simulink model "METI_Thermal_ver01_Jmaab_2018b_Intg"  (R2018b)
settings: Solver=ode8  StartTime=0  StopTime=end_time  FixedStep=sampling_time  RelTol=1e-3
PreLoadFcn:
  | %init_setting;
values from neighbouring files (symbols this model uses):
  degC2K = 273.15    [METI_TRAMI_Thermal_ver01_Jmaab_PreLoad.m]    (also in init_setting_METI.m)
  K2degC = -273.15    [METI_TRAMI_Thermal_ver01_Jmaab_PreLoad.m]    (also in init_setting_METI.m)
  sampling_time = 0.0025    [METI_TRAMI_Thermal_ver01_Jmaab_PreLoad.m]
undefined symbols (not defined in the file or in its folder): ACC_D_Gain, ACC_I_Gain, ACC_P_Gain, ALT_CNT_ALT_OFF_RPM_HYS_rpm, ALT_CNT_ALT_ON_RPM_HYS_rpm, ALT_CNT_Alter_V_BASE_V, ALT_CNT_Alter_V_Kaisei_V, ALT_CNT_flag_disable_kaisei, ALT_CNT_V_Battely_Kudo_V, ALT_PNT_ALT_GDCurrent_A, ALT_PNT_ALT_GDVolt_V, ALT_PNT_Alter_limit_Current_V_table, ALT_PNT_Alter_limit_Current_V_table_x_rpm, ALT_PNT_Alter_trq_Nm_map, ALT_PNT_Alter_trq_Nm_map_x_rpm, ALT_PNT_Alter_trq_Nm_map_y_Current_A, ALT_PNT_Alter_trq_Nm_map_z_Volt_tgt_V, ALT_PNT_eta_pulley_alt, ALT_PNT_Gain_Alt_v_del, ALT_PNT_ratio_pulley_alt, ALT_PNT_Tau_Alternator_V_tgt_s, ALT_PNT_trq_alter_output_LL_Nm, BK_PNT_Pow_UL, BK_PNT_Tau_brake, Brk_LL, Brk_PGain, Brk_UL, BT_PNT_Lo_Capa_lo_batt_F, BT_PNT_Lo_ocv_SOC_lo_batt_OCV_V_table, BT_PNT_Lo_ocv_SOC_lo_batt_OCV_V_table_x_SOC, BT_PNT_Lo_R_lo_batt_ohm, BT_PNT_Lo_SOC_MAX_lo_batt, BT_PNT_Lo_SOC_MIN_lo_batt, BT_PNT_Lo_SOC_START_lo_batt, BT_PNT_Lo_V_start_ocv, DF_PNT_DF_gear, DF_PNT_DFBlock2DFAir_Heat_Resi_KpW, DF_PNT_DFBlock_Heat_Capa_JpK, DF_PNT_DFBlock_Temp_ini_degC, DF_PNT_DFOil2DFBlock_Heat_Resi_KpW, DF_PNT_DFOil_Heat_Capa_JpK, DF_PNT_DFOil_Temp_ini_degC, DF_PNT_Driveshaft_damper, DF_PNT_Driveshaft_delta_radps_LL, DF_PNT_Driveshaft_delta_radps_UL, DF_PNT_Driveshaft_spring, DF_PNT_eta_DF, DF_PNT_Outtemp_degC, DF_PNT_TMBlock2DFBlock_Heat_Resi_KpW, Driver_Brake_Const1, Driver_Brake_Const3, Driver_Brake_Switch_Const2, Driver_Brk_sh, drivmode_ACC, drivmode_CONST, drivmode_GensokuKaisei, drivmode_GensokuRikko, drivmode_STOP, EL_PNT_R_bodyelec_lo_ohm, ENG_CNT_acc_idlestop ... (+137)
libraries: METI_Lib_vehicle_model x31, simulink x7, AZAPA_Lib_vehicle_model x1
(part 4 of 4)

== system METI_Thermal_ver01_Jmaab_2018b_Intg/Vehicle/PTTH/DTTH_PNT/DTTH_PNT/DFTH_PNT/TMBlock2DFBlock_Heat_Resistance ==
  T_DFBlock_Resi_K : Inport
  T_TMBlock_Resi_K : Inport  Port=2
  Add : Sum  Inputs=+-
  Constant : Constant  Value=DF_PNT_TMBlock2DFBlock_Heat_Resi_KpW
  Divide : Product  Inputs=*/
  Gain : Gain  Gain=-1
  Gain1 : Gain
  PHI_DFBlock_Resi_W : Outport
  PHI_TMBlock_Resi_W : Outport  Port=2
  wires:
  Constant/1 -> Divide/2
  Add/1 -> Divide/1
  Divide/1 -> Gain/1, Gain1/1
  Gain/1 -> PHI_TMBlock_Resi_W/1
  T_TMBlock_Resi_K/1 -> Add/1
  T_DFBlock_Resi_K/1 -> Add/2
  Gain1/1 -> PHI_DFBlock_Resi_W/1

== system METI_Thermal_ver01_Jmaab_2018b_Intg/Vehicle/PTTH/DTTH_PNT/DTTH_PNT/TMTH_PNT/CVTF2Coolant_Heat_Resistance ==
  note: エネルギーの
      | 向きの定義（仮）
      | ← ←←
  T_CVTF_Resi2_K : Inport
  R_CVTF_warmer_tgt_KpW : Inport  Port=2
  T_Coolant_Resi2_K : Inport  Port=3
  Add : Sum  Inputs=+-
  Divide : Product  Inputs=*/
  Gain : Gain  Gain=-1
  Gain1 : Gain  Gain=-1
  IC : InitialCondition  Value=0.1
  PHI_Coolant_Resi2_W : Outport
  PHI_CVTF_Resi2_W : Outport  Port=2
  wires:
  Add/1 -> Divide/1
  Divide/1 -> Gain/1, Gain1/1
  T_Coolant_Resi2_K/1 -> Add/2
  T_CVTF_Resi2_K/1 -> Add/1
  Gain/1 -> PHI_CVTF_Resi2_W/1
  Gain1/1 -> PHI_Coolant_Resi2_W/1
  IC/1 -> Divide/2
  R_CVTF_warmer_tgt_KpW/1 -> IC/1

== system METI_Thermal_ver01_Jmaab_2018b_Intg/Vehicle/PTTH/DTTH_PNT/DTTH_PNT/TMTH_PNT/CVTF2TMBlock_Heat_Resistance ==
  T_CVTF_Resi4_K : Inport
  T_TMBlock_Resi1_K : Inport  Port=2
  Add : Sum  Inputs=+-
  Constant : Constant  Value=TM_PNT_CVTF2TMBlock_Heat_Resi_KpW
  Divide : Product  Inputs=*/
  Gain : Gain  Gain=-1
  Gain1 : Gain
  PHI_CVTF_Resi4_W : Outport
  PHI_TMBlock_Resi1_W : Outport  Port=2
  wires:
  Constant/1 -> Divide/2
  Add/1 -> Divide/1
  Divide/1 -> Gain/1, Gain1/1
  Gain/1 -> PHI_CVTF_Resi4_W/1
  T_CVTF_Resi4_K/1 -> Add/1
  T_TMBlock_Resi1_K/1 -> Add/2
  Gain1/1 -> PHI_TMBlock_Resi1_W/1

== system METI_Thermal_ver01_Jmaab_2018b_Intg/Vehicle/PTTH/DTTH_PNT/DTTH_PNT/TMTH_PNT/CVTF_Heat_Capacity ==
  PHI_CVTF4_W : Inport
  PHI_CVTF1_W : Inport  Port=2
  PHI_CVT2_W : Inport  Port=3
  Add : Sum  Inputs=+++
  Add1 : Sum
  Constant : Constant  Value=TM_PNT_CVTF_Heat_Capa_JpK
  Constant1 : Constant  Value=TM_PNT_CVTF_Temp_ini_degC
  Divide : Product  Inputs=/*
  Integrator : Integrator
  degC->K : Subsystem
  T_CVTF4_K : Outport
  T_CVTF2_K : Outport  Port=2
  T_CVTF1_K : Outport  Port=3
  wires:
  PHI_CVT2_W/1 -> Add/3
  PHI_CVTF1_W/1 -> Add/1
  Constant/1 -> Divide/1
  Add/1 -> Divide/2
  Divide/1 -> Integrator/1
  Integrator/1 -> Add1/2
  Add1/1 -> T_CVTF1_K/1, T_CVTF2_K/1, T_CVTF4_K/1
  PHI_CVTF4_W/1 -> Add/2
  Constant1/1 -> degC->K/1(degC)
  degC->K/1(K) -> Add1/1

== system METI_Thermal_ver01_Jmaab_2018b_Intg/Vehicle/PTTH/DTTH_PNT/DTTH_PNT/TMTH_PNT/ENGBlock2TMBlock_Heat_Resistance ==
  T_TMBlock_Resi2_K : Inport
  T_ENGBlock_Resi2_K : Inport  Port=2
  Add : Sum  Inputs=+-
  Constant : Constant  Value=TM_PNT_ENGBlock2TMBlock_Heat_Resi_KpW
  Divide : Product  Inputs=*/
  Gain : Gain  Gain=-1
  Gain1 : Gain
  PHI_TMBlock_Resi2_W : Outport
  PHI_ENGBlock_Resi2_W : Outport  Port=2
  wires:
  Constant/1 -> Divide/2
  Add/1 -> Divide/1
  Divide/1 -> Gain1/1, Gain/1
  Gain/1 -> PHI_ENGBlock_Resi2_W/1
  T_ENGBlock_Resi2_K/1 -> Add/1
  T_TMBlock_Resi2_K/1 -> Add/2
  Gain1/1 -> PHI_TMBlock_Resi2_W/1

== system METI_Thermal_ver01_Jmaab_2018b_Intg/Vehicle/PTTH/DTTH_PNT/DTTH_PNT/TMTH_PNT/TMBlock2Air_Heat_Resistance ==
  T_TMBlock_Resi3_K : Inport
  T_TM_Air_Resi1_K : Inport  Port=2
  Add : Sum  Inputs=+-
  Constant : Constant  Value=TM_PNT_TMBlock2TMAir_Heat_Resi_KpW
  Divide : Product  Inputs=*/
  Gain : Gain  Gain=-1
  Gain1 : Gain
  PHI_TMBlock_Resi3_W : Outport
  PHI_TM_Air_Resi1_W : Outport  Port=2
  wires:
  Constant/1 -> Divide/2
  Add/1 -> Divide/1
  Divide/1 -> Gain/1, Gain1/1
  Gain/1 -> PHI_TMBlock_Resi3_W/1
  T_TMBlock_Resi3_K/1 -> Add/1
  T_TM_Air_Resi1_K/1 -> Add/2
  Gain1/1 -> PHI_TM_Air_Resi1_W/1

== system METI_Thermal_ver01_Jmaab_2018b_Intg/Vehicle/PTTH/DTTH_PNT/DTTH_PNT/TMTH_PNT/TMBlock_Heat_Capacity ==
  PHI_TMBlock3_W : Inport
  PHI_TMBlock2_W : Inport  Port=2
  PHI_TMBlock1_W : Inport  Port=3
  PHI_TMBlock4_W : Inport  Port=4
  Add : Sum  Inputs=++++
  Add1 : Sum
  Constant : Constant  Value=TM_PNT_TMBlock_Heat_Capa_JpK
  Constant1 : Constant  Value=TM_PNT_TMBlock_Temp_ini_degC
  Divide : Product  Inputs=/*
  Integrator : Integrator
  degC->K : Subsystem
  T_TMBlock2_K : Outport
  T_TMBlock3_K : Outport  Port=2
  T_TMBlock4_K : Outport  Port=3
  T_TMBlock1_K : Outport  Port=4
  wires:
  PHI_TMBlock2_W/1 -> Add/4
  PHI_TMBlock1_W/1 -> Add/1
  Constant/1 -> Divide/1
  Add/1 -> Divide/2
  Divide/1 -> Integrator/1
  Integrator/1 -> Add1/2
  PHI_TMBlock3_W/1 -> Add/3
  PHI_TMBlock4_W/1 -> Add/2
  Add1/1 -> T_TMBlock1_K/1, T_TMBlock4_K/1, T_TMBlock3_K/1, T_TMBlock2_K/1
  Constant1/1 -> degC->K/1(degC)
  degC->K/1(K) -> Add1/1

== system METI_Thermal_ver01_Jmaab_2018b_Intg/Vehicle/PTTH/ENGTH_PNT/ENGTH/Coolant_Heat_Capacity/degC->K ==
  degC : Inport
  Constant2 : Constant  Value=degC2K
  Sum : Sum  Inputs=++|
  K : Outport
  wires:
  degC/1 -> Sum/2
  Constant2/1 -> Sum/1
  Sum/1 -> K/1

== system METI_Thermal_ver01_Jmaab_2018b_Intg/Vehicle/PTTH/ENGTH_PNT/ENGTH/ENGBlock_Heat_Capacity/degC->K ==
  degC : Inport
  Constant2 : Constant  Value=degC2K
  Sum : Sum  Inputs=++|
  K : Outport
  wires:
  degC/1 -> Sum/2
  Constant2/1 -> Sum/1
  Sum/1 -> K/1

== system METI_Thermal_ver01_Jmaab_2018b_Intg/Vehicle/PTTH/ENGTH_PNT/ENGTH/ENGOil_Heat_Capacity/degC->K ==
  degC : Inport
  Constant2 : Constant  Value=degC2K
  Sum : Sum  Inputs=++|
  K : Outport
  wires:
  degC/1 -> Sum/2
  Constant2/1 -> Sum/1
  Sum/1 -> K/1

== system METI_Thermal_ver01_Jmaab_2018b_Intg/Vehicle/PTTH/ENGTH_PNT/ENGTH/ENGOil_Heat_Capacity1/degC->K ==
  degC : Inport
  Constant2 : Constant  Value=degC2K
  Sum : Sum  Inputs=++|
  K : Outport
  wires:
  degC/1 -> Sum/2
  Constant2/1 -> Sum/1
  Sum/1 -> K/1

== system METI_Thermal_ver01_Jmaab_2018b_Intg/Vehicle/PTTH/RDTH_PNT/RDTH/ENGBlock2Coolant_Heat_Resistance/K->degC ==
  K : Inport
  Constant2 : Constant  Value=K2degC
  Sum : Sum  Inputs=++|
  degC : Outport
  wires:
  K/1 -> Sum/2
  Constant2/1 -> Sum/1
  Sum/1 -> degC/1

== system METI_Thermal_ver01_Jmaab_2018b_Intg/Vehicle/PTTH/RDTH_PNT/RDTH/RDCoolant_Heat_Capacity/degC->K ==
  degC : Inport
  Constant2 : Constant  Value=degC2K
  Sum : Sum  Inputs=++|
  K : Outport
  wires:
  degC/1 -> Sum/2
  Constant2/1 -> Sum/1
  Sum/1 -> K/1

== system METI_Thermal_ver01_Jmaab_2018b_Intg/Vehicle/TM_PNT/TM_PNT/TM_PNT/TC_PNT/LU_Clutch ==
  note: クラッチモデル
      | LockUp ON時は硬いバネダンパー、OFF時はトルク0 Nm
  LockUP_Signal : Inport
  w_TM_PNT_in_radps1 : Inport  Port=2
  w_TM_PNT_in_radps2 : Inport  Port=3
  Gain1 : Gain  Gain=TM_PNT_Gain_LU_spring_Nmprad
  Gain2 : Gain  Gain=TM_PNT_Gain_LU_damper_Nmsprad
  Integrator : Integrator  ExternalReset=level  LimitOutput=on  UpperSaturationLimit=1  LowerSaturationLimit=-1
  Logical Operator : Logic  Operator=NOT  AllPortsSameDT=off  OutDataTypeStr=boolean
  Product : Product  RndMeth=Zero
  Product2 : Product  RndMeth=Zero
  Sum1 : Sum  Inputs=|+-
  Sum2 : Sum  Inputs=++|
  Transfer Fcn : TransferFcn  Denominator=[TM_PNT_tau_LU_Clutch_s 1]
  trq_LUC_Nm1 : Outport
  trq_LUC_Nm2 : Outport  Port=2
  wires:
  w_TM_PNT_in_radps1/1 -> Product/2
  LockUP_Signal/1 -> Logical Operator/1, Transfer Fcn/1
  Sum2/1 -> trq_LUC_Nm2/1, trq_LUC_Nm1/1
  Product2/1 -> Sum1/2
  Product/1 -> Sum1/1
  Integrator/1 -> Gain1/1
  Sum1/1 -> Integrator/1, Gain2/1
  Transfer Fcn/1 -> Product2/1, Product/1
  w_TM_PNT_in_radps2/1 -> Product2/2
  Logical Operator/1 -> Integrator/2
  Gain1/1 -> Sum2/2
  Gain2/1 -> Sum2/1

== system METI_Thermal_ver01_Jmaab_2018b_Intg/Vehicle/TM_PNT/TM_PNT/TM_PNT/TC_PNT/T_C ==
  w_TM_PNT_in_radps1 : Inport
  w_TM_PNT_in_radps2 : Inport  Port=2
  Cal_C_Capacity : Subsystem
  Cal_Ratio_n : Subsystem
  Cal_trq_TC_eng : Subsystem
  Gain : Gain  Gain=radpsec2rpm
  Gain1 : Gain  Gain=radpsec2rpm
  Product1 : Product  RndMeth=Zero
  トルク比 Lookup Table2 : Lookup_n-D  NumberOfTableDimensions=1  BreakpointsForDimension1=TM_PNT_torque_ratio_table_x_speed_ratio  Table=TM_PNT_torque_ratio_table  ExtrapMethod=Clip  RndMeth=Simplest  InputSameDT=on
  trq_TC_Nm1 : Outport
  trq_TC_Nm2 : Outport  Port=2
  wires:
  Gain/1 -> Cal_Ratio_n/2(n_GR_rpm)  "n_GR_rpm"
  Gain1/1 -> Cal_Ratio_n/1(n_TM_PNT_rpm), Cal_trq_TC_eng/1("n_TM_PNT_rpm ")  "n_TM_PNT_rpm"
  w_TM_PNT_in_radps2/1 -> Gain/1
  Product1/1 -> trq_TC_Nm1/1
  トルク比 Lookup Table2/1 -> Product1/2
  w_TM_PNT_in_radps1/1 -> Gain1/1
  Cal_Ratio_n/1(ratio_n) -> トルク比 Lookup Table2/1, Cal_C_Capacity/1(ratio_n)
  Cal_trq_TC_eng/1(trq_TC_Nm) -> trq_TC_Nm2/1, Product1/1  "trq_TC_Nm"
  Cal_C_Capacity/1(c_capacity) -> Cal_trq_TC_eng/2(c_capacity)
  Cal_Ratio_n/2(flag_acc_del) -> Cal_C_Capacity/2(flag_acc_del)

== system METI_Thermal_ver01_Jmaab_2018b_Intg/Vehicle/PTTH/DTTH_PNT/DTTH_PNT/DFTH_PNT/DFBlock_Heat_Capacity/degC->K ==
  degC : Inport
  Constant2 : Constant  Value=degC2K
  Sum : Sum  Inputs=++|
  K : Outport
  wires:
  degC/1 -> Sum/2
  Constant2/1 -> Sum/1
  Sum/1 -> K/1

== system METI_Thermal_ver01_Jmaab_2018b_Intg/Vehicle/PTTH/DTTH_PNT/DTTH_PNT/DFTH_PNT/DFOil_Heat_Capacity/degC->K ==
  degC : Inport
  Constant2 : Constant  Value=degC2K
  Sum : Sum  Inputs=++|
  K : Outport
  wires:
  degC/1 -> Sum/2
  Constant2/1 -> Sum/1
  Sum/1 -> K/1

== system METI_Thermal_ver01_Jmaab_2018b_Intg/Vehicle/PTTH/DTTH_PNT/DTTH_PNT/TMTH_PNT/CVTF_Heat_Capacity/degC->K ==
  degC : Inport
  Constant2 : Constant  Value=degC2K
  Sum : Sum  Inputs=++|
  K : Outport
  wires:
  degC/1 -> Sum/2
  Constant2/1 -> Sum/1
  Sum/1 -> K/1

== system METI_Thermal_ver01_Jmaab_2018b_Intg/Vehicle/PTTH/DTTH_PNT/DTTH_PNT/TMTH_PNT/TMBlock_Heat_Capacity/degC->K ==
  degC : Inport
  Constant2 : Constant  Value=degC2K
  Sum : Sum  Inputs=++|
  K : Outport
  wires:
  degC/1 -> Sum/2
  Constant2/1 -> Sum/1
  Sum/1 -> K/1

== system METI_Thermal_ver01_Jmaab_2018b_Intg/Vehicle/TM_PNT/TM_PNT/TM_PNT/TC_PNT/T_C/Cal_C_Capacity ==
  note: 容量係数
      | 加速中は＋
      | 減速中は－
  note: capacity coefficient
  note: N・m/rpm2
  ratio_n : Inport
  flag_acc_del : Inport  Port=2
  Product2 : Product  RndMeth=Zero
  ×10＾-6 : Gain  Gain=TM_PNT_ConvUnit
  容量係数 Lookup Table1 : Lookup_n-D  NumberOfTableDimensions=1  BreakpointsForDimension1=TM_PNT_torque_capacity_Nmprpm2_table_x_speed_ratio  Table=TM_PNT_torque_capacity_Nmprpm2_table  RndMeth=Simplest  InputSameDT=on
  c_capacity : Outport
  wires:
  容量係数 Lookup Table1/1 -> ×10＾-6/1
  ×10＾-6/1 -> Product2/1
  ratio_n/1 -> 容量係数 Lookup Table1/1
  Product2/1 -> c_capacity/1
  flag_acc_del/1 -> Product2/2

== system METI_Thermal_ver01_Jmaab_2018b_Intg/Vehicle/TM_PNT/TM_PNT/TM_PNT/TC_PNT/T_C/Cal_Ratio_n ==
  n_TM_PNT_rpm : Inport
  n_GR_rpm : Inport  Port=2
  Compare To Constant1 : simulink/Logic and Bit Operations/Compare To Constant  relop=<=  const=TM_PNT_n_TC_min_rpm  OutDataTypeStr=boolean
  Compare To Constant2 : simulink/Logic and Bit Operations/Compare To Constant  relop=<=  const=TM_PNT_n_TC_min_rpm  OutDataTypeStr=boolean
  Constant : Constant  Value=0
  Logical Operator1 : Logic  Operator=OR  AllPortsSameDT=off  OutDataTypeStr=boolean
  MinMax : MinMax  Inputs=2
  Saturation1 : Saturate  UpperLimit=TM_PNT_w_ROT_T_C_UL  LowerLimit=TM_PNT_w_ROT_T_C_LL
  Saturation2 : Saturate  UpperLimit=TM_PNT_w_ROT_T_C_UL  LowerLimit=TM_PNT_w_ROT_T_C_LL
  Saturation5 : Saturate  UpperLimit=TM_PNT_ratio_w_ROT_T_C_UL  LowerLimit=TM_PNT_ratio_w_ROT_T_C_LL
  Subsystem : Subsystem
  Switch : Switch  Threshold=0.5
  加速時速度比 : Product  Inputs=*/
  減速時速度比 : Product  Inputs=*/
  ratio_n : Outport
  flag_acc_del : Outport  Port=2
  wires:
  Saturation2/1 -> 減速時速度比/1, 加速時速度比/2
  Saturation1/1 -> 減速時速度比/2, 加速時速度比/1
  加速時速度比/1 -> MinMax/1
  減速時速度比/1 -> MinMax/2
  MinMax/1 -> Saturation5/1
  Saturation5/1 -> Switch/3
  Constant/1 -> Switch/1
  Compare To Constant2/1 -> Logical Operator1/1
  Compare To Constant1/1 -> Logical Operator1/2
  Logical Operator1/1 -> Switch/2
  Switch/1 -> ratio_n/1
  n_GR_rpm/1 -> Subsystem/2(omg_tm), Saturation1/1, Compare To Constant1/1  "omg_tm"
  n_TM_PNT_rpm/1 -> Compare To Constant2/1, Subsystem/1(omg_engine), Saturation2/1  "omg_engine"
  Subsystem/1(flag_acc_del) -> flag_acc_del/1

== system METI_Thermal_ver01_Jmaab_2018b_Intg/Vehicle/TM_PNT/TM_PNT/TM_PNT/TC_PNT/T_C/Cal_trq_TC_eng ==
  "n_TM_PNT_rpm " : Inport
  c_capacity : Inport  Port=2
  Math Function : Math  Operator=magnitude^2  SaturateOnIntegerOverflow=on
  Product : Product  RndMeth=Zero
  trq_TC_Nm : Outport
  wires:
  Product/1 -> trq_TC_Nm/1
  Math Function/1 -> Product/1
  c_capacity/1 -> Product/2
  "n_TM_PNT_rpm "/1 -> Math Function/1

== system METI_Thermal_ver01_Jmaab_2018b_Intg/Vehicle/TM_PNT/TM_PNT/TM_PNT/TC_PNT/T_C/Cal_Ratio_n/Subsystem ==
  note: エンジン加速中は1、減速中は-1
  omg_engine : Inport
  omg_tm : Inport  Port=2
  Saturation : Saturate  UpperLimit=1  LowerLimit=-1
  Subtract : Sum  Inputs=-+|
  flag_acc_del : Outport
  wires:
  Subtract/1 -> Saturation/1
  Saturation/1 -> flag_acc_del/1
  omg_tm/1 -> Subtract/1
  omg_engine/1 -> Subtract/2
